simulink model "MultirotorSimPx4v1_8TuningRateCont"  (R2020b)
settings: Solver=VariableStepAuto  StartTime=0.0  StopTime=Simulation.T_END  MaxStep=Simulation.TS_MAX  RelTol=1e-3  EnableMultiTasking=on
PreLoadFcn:
  | % InitializeParameters;
undefined symbols (not defined in the file): DiscIntNeverNeededParam, Initial, Simulation, Uav, Wind
libraries: QuaternionLibrary x10, simulink x3, simulink_extras x2
(part 2 of 2)

== matlab function MultirotorSimPx4v1_8TuningRateCont/Applied wind speed/Relative velocity ==
  data: nuBody input; Uav parameter; VMotorRelBody output
function VMotorRelBody = relativeMotorVelocity( nuBody , Uav )
%#codegen
    VMotorRelBody = cross( nuBody, Uav.L_VEC );
end

== matlab function MultirotorSimPx4v1_8TuningRateCont/Applied wind speed/Compute V_app2 ==
  data: Q input; UBody output; U input size=3
function UBody = computeUBody(Q, U)
%#codegen

% Rotation matrix from Wind frame to Inertial frame
% Wind frame SEU, inertial frame NED
R_U = [1,  0, 0;
       0, -1, 0;
       0,  0, 1];
   
UBody = Q' * R_U * U;

== matlab function MultirotorSimPx4v1_8TuningRateCont/Attitude Controller/Filter ==
  data: input input; self input; output output; self output
function [ output, self ] = Filter( input, self )
    % 'Decode' self vector
    obj.lp_filters_d_a1 = self(1);
    obj.lp_filters_d_a2 = self(2);
    obj.lp_filters_d_b0 = self(3);
    obj.lp_filters_d_b1 = self(4);
    obj.lp_filters_d_b2 = self(5);
    obj.lp_filters_d_cutoff_freq = 30;
    obj.lp_filters_d_delay_element_1 = self(7:9);
    obj.lp_filters_d_delay_element_2 = self(10:12);
    init = self(13);
    
    % Variables
    sample_freq = 250;
    cutoff_freq = 30;
    
    if ~init
        obj = LowPassFilter2pVectorSetCutOffFrequency( obj, sample_freq, cutoff_freq );
        init = 1;
    end
    
    [obj, output] = LowPassFilter2pVector3Apply( obj, input );

    % 'Encode' self vector
    self(1)     = obj.lp_filters_d_a1;
    self(2)     = obj.lp_filters_d_a2;
    self(3)     = obj.lp_filters_d_b0;
    self(4)     = obj.lp_filters_d_b1;
    self(5)     = obj.lp_filters_d_b2;
    self(6)     = obj.lp_filters_d_cutoff_freq;
    self(7:9)    = obj.lp_filters_d_delay_element_1;
    self(10:12) = obj.lp_filters_d_delay_element_2;
    self(13) = init;
end

function [obj, output] = LowPassFilter2pVector3Apply( obj, sample )
    %LOWPASSFILTER2PVECTOR3APPLY Apply low pass filter
    %   Based on code from PX4 Firmware:
    %       https://github.com/PX4/Firmware/blob/master/src/lib/mathlib/math/filter/LowPassFilter2pVector3f.hpp
    %   Written:       J.X.J. Bannwarth, 2019/01/16
    %   Last modified: J.X.J. Bannwarth, 2019/01/21
    delay_element_0 = sample - obj.lp_filters_d_delay_element_1.*obj.lp_filters_d_a1 - obj.lp_filters_d_delay_element_2.*obj.lp_filters_d_a2;
    output = delay_element_0.*obj.lp_filters_d_b0 + obj.lp_filters_d_delay_element_1.*obj.lp_filters_d_b1 + obj.lp_filters_d_delay_element_2*obj.lp_filters_d_b2;
    obj.lp_filters_d_delay_element_2 = obj.lp_filters_d_delay_element_1;
    obj.lp_filters_d_delay_element_1 = delay_element_0;
end

    function obj =  LowPassFilter2pVectorSetCutOffFrequency( obj, sample_freq, cutoff_freq )
    %LOWPASSFILTER2PVECTOR3SETCUTOFFFREQUENCY Set cutoff frequency
    %   Based on code from PX4 Firmware:
    %       https://github.com/PX4/Firmware/blob/master/src/lib/mathlib/math/filter/LowPassFilter2pVector3f.cpp
    %   Written:       J.X.J. Bannwarth, 2019/01/16
    %   Last modified: J.X.J. Bannwarth, 2019/01/21
    obj.lp_filters_d_cutoff_freq = cutoff_freq;

    % Reset delay elements on filter change
    obj.lp_filters_d_delay_element_1 = zeros(3,1);
    obj.lp_filters_d_delay_element_2 = zeros(3,1);

    if (obj.lp_filters_d_cutoff_freq <= 0.0)
        % No filtering
        obj.lp_filters_d_b0 = 1.0;
        obj.lp_filters_d_b1 = 0.0;
        obj.lp_filters_d_b2 = 0.0;

        obj.lp_filters_d_a1 = 0.0;
        obj.lp_filters_d_a2 = 0.0;
        return
    end

    fr = sample_freq / obj.lp_filters_d_cutoff_freq;
    ohm = tan( pi / fr);
    c = 1.0 + 2.0 * cos( pi / 4.0) * ohm + ohm * ohm;

    obj.lp_filters_d_b0 = ohm * ohm / c;
    obj.lp_filters_d_b1 = 2.0 * obj.lp_filters_d_b0;
    obj.lp_filters_d_b2 = obj.lp_filters_d_b0;

    obj.lp_filters_d_a1 = 2.0 * (ohm * ohm - 1.0) / c;
    obj.lp_filters_d_a2 = (1.0 - 2.0 * cos(pi / 4.0) * ohm + ohm * ohm) / c;
end

% function output = LowPassFilter2pVectorReset( obj, sample )
%     %LOWPASSFILTER2PVECTOR3SETCUTOFFFREQUENCY Set cutoff frequency
%     %   Based on code from PX4 Firmware:
%     %       https://github.com/PX4/Firmware/blob/master/src/lib/mathlib/math/filter/LowPassFilter2pVector3f.cpp
%     %   Written:       J.X.J. Bannwarth, 2019/01/16
%     %   Last modified: J.X.J. Bannwarth, 2019/01/21
%     dval = sample ./ (obj.lp_filters_d_b0 + obj.lp_filters_d_b1 + obj.lp_filters_d_b2);
% 
%     if (isfinite( dval(1) ) && isfinite( dval(2) ) && isfinite( dval(3) ))
%         obj.lp_filters_d_delay_element_1 = dval;
%         obj.lp_filters_d_delay_element_2 = dval;
%     else
%         obj.lp_filters_d_delay_element_1 = sample;
%         obj.lp_filters_d_delay_element_2 = sample;
%     end
% 
%     output = LowPassFilter2pVector3Apply( obj, sample );
% end

== matlab function MultirotorSimPx4v1_8TuningRateCont/Attitude Controller/MATLAB Function ==
  data: input input; self input; output output; self output
function [ output, self ] = Filter( input, self )
    % 'Decode' self vector
    obj.lp_filters_d_a1 = self(1);
    obj.lp_filters_d_a2 = self(2);
    obj.lp_filters_d_b0 = self(3);
    obj.lp_filters_d_b1 = self(4);
    obj.lp_filters_d_b2 = self(5);
    obj.lp_filters_d_cutoff_freq = self(6);
    obj.lp_filters_d_delay_element_1 = self(7:9);
    obj.lp_filters_d_delay_element_2 = self(10:12);
    init = self(13);
    
    % Variables
    sample_freq = 250;
    cutoff_freq = 30;
    
    if ~init
        obj = LowPassFilter2pVectorSetCutOffFrequency( obj, sample_freq, cutoff_freq );
        init = 1;
    end
    
    [obj, output] = LowPassFilter2pVector3Apply( obj, input );

    % 'Encode' self vector
    self(1)     = obj.lp_filters_d_a1;
    self(2)     = obj.lp_filters_d_a2;
    self(3)     = obj.lp_filters_d_b0;
    self(4)     = obj.lp_filters_d_b1;
    self(5)     = obj.lp_filters_d_b2;
    self(6)     = obj.lp_filters_d_cutoff_freq;
    self(7:9)    = obj.lp_filters_d_delay_element_1;
    self(10:12) = obj.lp_filters_d_delay_element_2;
    self(13) = init;
end

function [obj, output] = LowPassFilter2pVector3Apply( obj, sample )
    %LOWPASSFILTER2PVECTOR3APPLY Apply low pass filter
    %   Based on code from PX4 Firmware:
    %       https://github.com/PX4/Firmware/blob/master/src/lib/mathlib/math/filter/LowPassFilter2pVector3f.hpp
    %   Written:       J.X.J. Bannwarth, 2019/01/16
    %   Last modified: J.X.J. Bannwarth, 2019/01/21
    delay_element_0 = sample - obj.lp_filters_d_delay_element_1.*obj.lp_filters_d_a1 - obj.lp_filters_d_delay_element_2.*obj.lp_filters_d_a2;
    output = delay_element_0.*obj.lp_filters_d_b0 + obj.lp_filters_d_delay_element_1.*obj.lp_filters_d_b1 + obj.lp_filters_d_delay_element_2*obj.lp_filters_d_b2;
    obj.lp_filters_d_delay_element_2 = obj.lp_filters_d_delay_element_1;
    obj.lp_filters_d_delay_element_1 = delay_element_0;
end

    function obj =  LowPassFilter2pVectorSetCutOffFrequency( obj, sample_freq, cutoff_freq )
    %LOWPASSFILTER2PVECTOR3SETCUTOFFFREQUENCY Set cutoff frequency
    %   Based on code from PX4 Firmware:
    %       https://github.com/PX4/Firmware/blob/master/src/lib/mathlib/math/filter/LowPassFilter2pVector3f.cpp
    %   Written:       J.X.J. Bannwarth, 2019/01/16
    %   Last modified: J.X.J. Bannwarth, 2019/01/21
    obj.lp_filters_d_cutoff_freq = cutoff_freq;

    % Reset delay elements on filter change
    obj.lp_filters_d_delay_element_1 = zeros(3,1);
    obj.lp_filters_d_delay_element_2 = zeros(3,1);

    if (obj.lp_filters_d_cutoff_freq <= 0.0)
        % No filtering
        obj.lp_filters_d_b0 = 1.0;
        obj.lp_filters_d_b1 = 0.0;
        obj.lp_filters_d_b2 = 0.0;

        obj.lp_filters_d_a1 = 0.0;
        obj.lp_filters_d_a2 = 0.0;
        return
    end

    fr = sample_freq / obj.lp_filters_d_cutoff_freq;
    ohm = tan( pi / fr);
    c = 1.0 + 2.0 * cos( pi / 4.0) * ohm + ohm * ohm;

    obj.lp_filters_d_b0 = ohm * ohm / c;
    obj.lp_filters_d_b1 = 2.0 * obj.lp_filters_d_b0;
    obj.lp_filters_d_b2 = obj.lp_filters_d_b0;

    obj.lp_filters_d_a1 = 2.0 * (ohm * ohm - 1.0) / c;
    obj.lp_filters_d_a2 = (1.0 - 2.0 * cos(pi / 4.0) * ohm + ohm * ohm) / c;
end

% function output = LowPassFilter2pVectorReset( obj, sample )
%     %LOWPASSFILTER2PVECTOR3SETCUTOFFFREQUENCY Set cutoff frequency
%     %   Based on code from PX4 Firmware:
%     %       https://github.com/PX4/Firmware/blob/master/src/lib/mathlib/math/filter/LowPassFilter2pVector3f.cpp
%     %   Written:       J.X.J. Bannwarth, 2019/01/16
%     %   Last modified: J.X.J. Bannwarth, 2019/01/21
%     dval = sample ./ (obj.lp_filters_d_b0 + obj.lp_filters_d_b1 + obj.lp_filters_d_b2);
% 
%     if (isfinite( dval(1) ) && isfinite( dval(2) ) && isfinite( dval(3) ))
%         obj.lp_filters_d_delay_element_1 = dval;
%         obj.lp_filters_d_delay_element_2 = dval;
%     else
%         obj.lp_filters_d_delay_element_1 = sample;
%         obj.lp_filters_d_delay_element_2 = sample;
%     end
% 
%     output = LowPassFilter2pVector3Apply( obj, sample );
% end

== matlab function MultirotorSimPx4v1_8TuningRateCont/Compute Sph ==
  data: in input; beta output; alpha output; R output
function [beta, alpha, R] = computeSph(in)
%#codegen

% Convert from polar to spherical coordinates
[ beta, alpha, R ] = cart2sph( in(1), in(2), in(3) );
